simulink library "crm_grc"  (R2024a)
settings: Solver=VariableStepAuto  StartTime=0.0  StopTime=10.0  RelTol=1e-3
undefined symbols (not defined in the file or in its folder): ACRM_Eta_X_rpm, ACRM_MTPAIdGen_X_rpm, ACRM_MTPAIdGen_Y_Nm, ACRM_MTPAIdGenMin_X_rpm, ACRM_MTPAIdGenMin_Y_Nm, ACRM_MTPAIdMot_X_rpm, ACRM_MTPAIdMot_Y_Nm, ACRM_MTPAIdMotMin_X_rpm, ACRM_MTPAIdMotMin_Y_Nm, ACRM_MTPAIqGen_X_rpm, ACRM_MTPAIqGen_Y_Nm, ACRM_MTPAIqGenMin_X_rpm, ACRM_MTPAIqGenMin_Y_Nm, ACRM_MTPAIqMot_X_rpm, ACRM_MTPAIqMot_Y_Nm, ACRM_MTPAIqMotMin_X_rpm, ACRM_MTPAIqMotMin_Y_Nm, ACRM_MTPVIdLimt_X_rpm, DiscIntNeverNeededParam, ENUM_MOTMOD_DISCHARGE, GRC_FAKE_SAMPLE_TIME, KCRM_AtSweep_deg_ovrdflg, KCRM_AtSweep_deg_ovrdval, KCRM_AtSwFWThd_V, KCRM_AtSwStep_ms, KCRM_AtSwThetaStep_deg, KCRM_bRstDebugOverSpd_null, KCRM_BusCurFil_null, KCRM_CurDebugSwt_null, KCRM_CurTqCmdHi_Nm, KCRM_CurTqCmdLo_Nm, KCRM_DcHiBatLDerat_V, KCRM_DcHiBatLLim_V, KCRM_DynoDeratingFiltFac_null, KCRM_FWCEnable_null, KCRM_FWCKi_null, KCRM_FWCKp_null, KCRM_grdIsThetaRampDown_C, KCRM_grdIsThetaRampUp_C, KCRM_IdCmdFilCoeff_null, KCRM_IdCmdMaxLimt_A, KCRM_IdqMapVolHi_V, KCRM_IdqMapVolLo_V, KCRM_IdSp_A_ovrdval, KCRM_IdSpForActvDisc_null, KCRM_IqCmdFilCoeff_null, KCRM_IqDeratingFac_null, KCRM_IqDeratingRecoverTi_ms, KCRM_IqDeratingTi_ms, KCRM_IqDerForFluxWeaken_fac, KCRM_IqSp_A_ovrdval, KCRM_IsSp_A, KCRM_MinVolOfst4FW_V, KCRM_MTPAGenSwitch_flg, KCRM_MTPAMotSwitch_flg, KCRM_MTPVSpdThd_rpm, KCRM_nDebugOverSpd_rpm, KCRM_OCSwFltNormThd_A, KCRM_PILowerLimit_null, KCRM_SpdCtlPrd_s ... (+24)
libraries: GRC_Lib x5, simulink x4
(part 2 of 2)

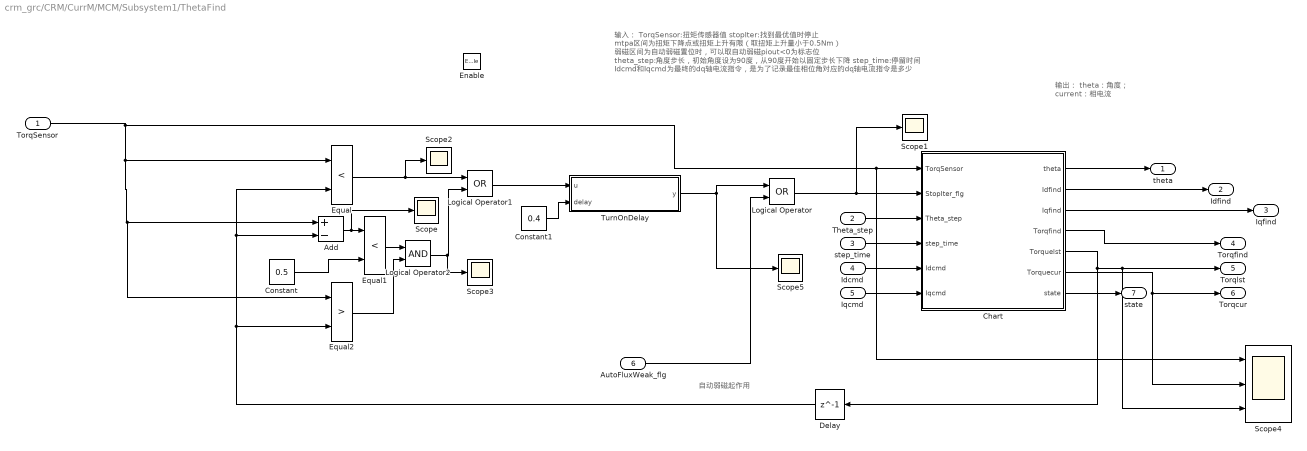
== system crm_grc/CRM/CurrM/MCM/Subsystem1/ThetaFind ==
  note: 输出：
      | theta：角度；
      | current：相电流
  note: 输入：
      | TorqSensor:扭矩传感器值
      | stopIter:找到最优值时停止 mtpa区间为扭矩下降点或扭矩上升有限（取扭矩上升量小于0.5Nm） 弱磁区间为自动弱磁置位时，可以取自动弱磁piout<0为标志位
      | theta_step:角度步长，初始角度设为90度，从90度开始以固定步长下降
      | step_time:停留时间
      | Idcmd和Iqcmd为最终的dq轴电流指令，是为了记录最佳相位角对应的dq轴电流指令是多少
  note: 自动弱磁起作用
  TorqSensor : Inport
  Theta_step : Inport  Port=2
  step_time : Inport  Port=3
  Idcmd : Inport  Port=4
  Iqcmd : Inport  Port=5
  AutoFluxWeak_flg : Inport  Port=6
  Enable : EnablePort  StatesWhenEnabling=reset
  Add : Sum  Inputs=+-
  Chart : Stateflow chart  TreatAsAtomicUnit=on
  Constant : Constant  Value=0.5
  Constant1 : Constant  Value=0.4  OutDataTypeStr=single
  Delay : Delay  DelayLength=1  InputProcessing=Columns as channels (frame based)
  Equal : RelationalOperator  Operator=<  OutDataTypeStr=boolean  RndMeth=Simplest  InputSameDT=off
  Equal1 : RelationalOperator  Operator=<  OutDataTypeStr=boolean  RndMeth=Simplest  InputSameDT=off
  Equal2 : RelationalOperator  Operator=>  OutDataTypeStr=boolean  RndMeth=Simplest  InputSameDT=off
  Logical Operator : Logic  Operator=OR  AllPortsSameDT=off  OutDataTypeStr=boolean
  Logical Operator1 : Logic  Operator=OR  AllPortsSameDT=off  OutDataTypeStr=boolean
  Logical Operator2 : Logic  AllPortsSameDT=off  OutDataTypeStr=boolean
  Scope{,1..3,5} (5 alike) : Scope
  Scope4 : Scope  NumInputPorts=3
  TurnOnDelay : Subsystem  AncestorBlock=Legion_lib/Logic Blocks/TurnOnDelay
      mask Display:
      | color('red');
      | disp('Turn On Delay')
  theta : Outport  VectorParamsAs1DForOutWhenUnconnected=off
  Idfind : Outport  Port=2  VectorParamsAs1DForOutWhenUnconnected=off
  Iqfind : Outport  Port=3  VectorParamsAs1DForOutWhenUnconnected=off
  Torqfind : Outport  Port=4  VectorParamsAs1DForOutWhenUnconnected=off
  Torqlst : Outport  Port=5  VectorParamsAs1DForOutWhenUnconnected=off
  Torqcur : Outport  Port=6  VectorParamsAs1DForOutWhenUnconnected=off
  state : Outport  Port=7  VectorParamsAs1DForOutWhenUnconnected=off
  wires:
  Constant1/1 -> TurnOnDelay/2(delay)
  TurnOnDelay/1(y) -> Logical Operator/1, Scope5/1
  Logical Operator1/1 -> TurnOnDelay/1(u)
  Chart/7(state) -> state/1
  Chart/6(Torquecur) -> Torqcur/1, Scope4/2
  Delay/1 -> Equal/2, Add/2, Equal2/2
  Chart/5(Torquelst) -> Torqlst/1, Scope4/3, Delay/1
  Logical Operator2/1 -> Logical Operator1/2, Scope3/1
  Equal2/1 -> Logical Operator2/2
  Equal1/1 -> Logical Operator2/1
  Constant/1 -> Equal1/2
  Add/1 -> Equal1/1, Scope/1
  Chart/4(Torqfind) -> Torqfind/1
  Equal/1 -> Logical Operator1/1, Scope2/1
  AutoFluxWeak_flg/1 -> Logical Operator/2
  Iqcmd/1 -> Chart/6(Iqcmd)
  Idcmd/1 -> Chart/5(Idcmd)
  Chart/3(Iqfind) -> Iqfind/1
  Chart/2(Idfind) -> Idfind/1
  Chart/1(theta) -> theta/1
  TorqSensor/1 -> Chart/1(TorqSensor), Scope4/1, Add/1, Equal2/1, Equal/1
  Theta_step/1 -> Chart/3(Theta_step)
  Logical Operator/1 -> Chart/2(StopIter_flg), Scope1/1
  step_time/1 -> Chart/4(step_time)

== system crm_grc/CRM/CurrM/MCM/FluxWeaken /PI /Anti-windup ==
  preInt : Inport
  preSat : Inport  Port=2
  Upper Limit : Inport  Port=3
  Lower Limit : Inport  Port=4
  AND3 : Logic  DisableCoverage=on  OutDataTypeStr=boolean
  Constant : Constant  DisableCoverage=on  OutDataTypeStr=int8
  Constant1 : Constant  DisableCoverage=on  Value=0  OutDataTypeStr=Inherit: Inherit via back propagation  PreserveConstantTs=on
  Constant2 : Constant  DisableCoverage=on  Value=-1  OutDataTypeStr=int8
  Constant3 : Constant  DisableCoverage=on  OutDataTypeStr=int8
  Constant4 : Constant  DisableCoverage=on  Value=-1  OutDataTypeStr=int8
  Constant5 : Constant  Value=0  OutDataTypeStr=Inherit: Inherit via back propagation
  Dead Zone Dynamic : simulink/Discontinuities/Dead Zone Dynamic
  Equal1 : RelationalOperator  DisableCoverage=on  Operator===  OutDataTypeStr=boolean  RndMeth=Simplest  InputSameDT=off
  Relational Operator : RelationalOperator  DisableCoverage=on  Operator=~=  OutDataTypeStr=boolean  RndMeth=Simplest  InputSameDT=off
  Relational Operator1 : RelationalOperator  Operator=>  OutDataTypeStr=boolean  RndMeth=Simplest  InputSameDT=off
  Relational Operator2 : RelationalOperator  Operator=>  OutDataTypeStr=boolean  RndMeth=Simplest  InputSameDT=off
  Switch1 : Switch  DisableCoverage=on  Criteria=u2 > Threshold  SaturateOnIntegerOverflow=off  InputSameDT=off
  Switch2 : Switch  DisableCoverage=on  Criteria=u2 > Threshold  SaturateOnIntegerOverflow=off  InputSameDT=off
  Switch3 : Switch  Criteria=u2 ~= 0  RndMeth=Simplest  SaturateOnIntegerOverflow=off  InputSameDT=off
  Out : Outport
  wires:
  Relational Operator2/1 -> Switch2/2
  Constant3/1 -> Switch2/1
  Constant4/1 -> Switch2/3
  AND3/1 -> Switch3/2  "VFWC_IntSat_flg"
  Relational Operator1/1 -> Switch1/2
  Constant2/1 -> Switch1/3
  Dead Zone Dynamic/1 -> Relational Operator/2, Relational Operator1/1
  Upper Limit/1 -> Dead Zone Dynamic/1
  Constant/1 -> Switch1/1
  Switch1/1 -> Equal1/1
  Switch2/1 -> Equal1/2
  Relational Operator/1 -> AND3/1
  preInt/1 -> Switch3/3, Relational Operator2/1
  Switch3/1 -> Out/1
  Constant5/1 -> Relational Operator2/2, Relational Operator1/2, Relational Operator/1
  Equal1/1 -> AND3/2
  preSat/1 -> Dead Zone Dynamic/2
  Lower Limit/1 -> Dead Zone Dynamic/3
  Constant1/1 -> Switch3/1

== system crm_grc/CRM/CurrM/MCM/Subsystem/ThetaFind/TurnOnDelay ==
  u : Inport
  delay : Inport  Port=2
  Data Type Conversion : DataTypeConversion  OutDataTypeStr=single  SaturateOnIntegerOverflow=off  RndMeth=Floor
  sample time : SampleTimeMath  TsampMathOp=Ts Only  weightValue=1  OutDataTypeStr=Inherit: Inherit via back propagation
  turnondelay : Stateflow chart  TreatAsAtomicUnit=on
  y : Outport
  wires:
  sample time/1 -> turnondelay/3(step)
  Data Type Conversion/1 -> sample time/1
  turnondelay/1(y) -> y/1
  delay/1 -> turnondelay/2(delay)
  u/1 -> Data Type Conversion/1, turnondelay/1(u)

== system crm_grc/CRM/CurrM/MCM/Subsystem1/ThetaFind/TurnOnDelay ==
  u : Inport
  delay : Inport  Port=2
  Data Type Conversion : DataTypeConversion  OutDataTypeStr=single  SaturateOnIntegerOverflow=off  RndMeth=Floor
  sample time : SampleTimeMath  TsampMathOp=Ts Only  weightValue=1  OutDataTypeStr=Inherit: Inherit via back propagation
  turnondelay : Stateflow chart  TreatAsAtomicUnit=on
  y : Outport
  wires:
  u/1 -> turnondelay/1(u), Data Type Conversion/1
  delay/1 -> turnondelay/2(delay)
  turnondelay/1(y) -> y/1
  Data Type Conversion/1 -> sample time/1
  sample time/1 -> turnondelay/3(step)

== stateflow chart crm_grc/CRM/CurrM/MCM/Subsystem/ThetaFind/TurnOnDelay/turnondelay ==
  state Off
    en:y=0;
    timer=0;
  state Delay
    en:timer=timer+step;
    du:timer=timer+step;
  state On
    en:y=1;
  (default) -> Off
  (junction 28) -> Off
  (junction 29) -> (junction 28)
  Delay -> Off [order 1] : [~u]
  Off -> (junction 17) : [u]
  (junction 17) -> (junction 24) [order 1] : [timer>=delay-10^-5]
  (junction 17) -> Delay [order 2]
  (junction 24) -> (junction 25)
  Delay -> On [order 2] : [timer>=delay-10^-5]
  On -> (junction 29) : [~u]
  (junction 25) -> On
  data: u input boolean; delay input single; y output boolean =0; timer local single =0; step input single

== stateflow chart crm_grc/CRM/CurrM/MCM/Subsystem1/ThetaFind/Chart ==
  state degression
    en:
    state = 2;
    theta = theta -Theta_step;
  state INIT
    en:
    theta = 80;
    state = 1;
    Torquelst=-5;
    Torquecur=TorqSensor;
  state end
    en:
    state = 4;
    Idfind = Idcmd;
    Iqfind = Iqcmd;
    theta = 90;
    Torqfind=TorqSensor;
  state wait1
    en:
    state = 3;
    du: cnt = cnt + 1;
  (default) -> INIT
  INIT -> degression
  degression -> wait1 : [theta >=0]{cnt = 0;}
  wait1 -> degression [order 2] : [cnt >= step_time]{cnt = 0;Torquecur=TorqSensor;Torquelst=Torquecur;}
  wait1 -> end [order 1] : [StopIter_flg]
  data: TorqSensor input; StopIter_flg input; Theta_step input; cnt local int32; theta output; step_time input; Idcmd input; Idfind output; Iqfind output; Torqfind output; Torquelst output; Iqcmd input; Torquecur output; state output int8

== stateflow chart crm_grc/CRM/CurrM/MCM/Subsystem1/ThetaFind/TurnOnDelay/turnondelay ==
  state Off
    en:y=0;
    timer=0;
  state Delay
    en:timer=timer+step;
    du:timer=timer+step;
  state On
    en:y=1;
  (default) -> Off
  (junction 28) -> Off
  (junction 29) -> (junction 28)
  Delay -> Off [order 1] : [~u]
  Off -> (junction 17) : [u]
  (junction 17) -> (junction 24) [order 1] : [timer>=delay-10^-5]
  (junction 17) -> Delay [order 2]
  (junction 24) -> (junction 25)
  Delay -> On [order 2] : [timer>=delay-10^-5]
  On -> (junction 29) : [~u]
  (junction 25) -> On
  data: u input boolean; delay input single; y output boolean =0; timer local single =0; step input single

== stateflow chart crm_grc/CRM/CurrM/MCM/IArb ==
  settings: description=$TL$ stepfunctionclass=GlobalFunctionClasses/INLINE_FCN; $TL$
  (default) -> (junction 32)
  (junction 32) -> (junction 35) [order 1] : [ActvDichEna_flg]
  (junction 32) -> (junction 11) [order 2]
  (junction 35) -> (junction 36) : {
      |   IdCmd = IdCmdForActvDich_A;
      |   IqCmd = 0;
      |  }
  (junction 11) -> (junction 12) [order 1] : [CurSpEna_flg]
  (junction 11) -> (junction 14) [order 2]
  (junction 12) -> (junction 13) : {
      |   IdCmd = IdSpAct;
      |   IqCmd = IqSpAct;
      |  }
  (junction 14) -> (junction 15) [order 1] : [CurLoopEna_flg]
  (junction 14) -> (junction 17) [order 2] : {
      |   IdCmd = 0;
      |   IqCmd = 0;
      |  }
  (junction 15) -> (junction 16) : {
      |   IdCmd = IdRef;
      |   IqCmd = IqRef;
      |  }
  (junction 16) -> (junction 17)
  (junction 13) -> (junction 16)
  (junction 36) -> (junction 13)
  (junction 17) -> (junction 18)
  data: IdRef input; IqRef input; IdSpAct input; IqSpAct input; CurLoopEna_flg input; IdCmd output single; IqCmd output single; CurSpEna_flg input boolean; ActvDichEna_flg input boolean; IdCmdForActvDich_A input single
  data IdRef settings: description=|
      | Current reference of d axis deduced by T-n
      | $TL$ variable=GLOBAL/LocalVariables/TM/Current/Id_Ref; $TL$
  data IqRef settings: description=|
      | Current reference of q axis deduced by T-n
      | $TL$ variable=GLOBAL/LocalVariables/TM/Current/Iq_Ref; $TL$
  data IdSpAct settings: description=|
      | Current setpoint of d axis
      | $TL$ variable=GLOBAL/GlobalVariables/MCU/Function/TM/APPL_TM_Id_Setp; $TL$
  data IqSpAct settings: description=|
      | Current setpoint of q axis
      | 
      | $TL$ variable=GLOBAL/GlobalVariables/MCU/Function/TM/APPL_TM_Iq_Setp; $TL$
  data CurLoopEna_flg settings: description=|
      | Control mode of TM controller, 0 for Voltage loop, 1 for Current loop, 2 for Torque loop, 3 for Speed loop
      | $TL$ variable=GLOBAL/GlobalVariables/MCU/Function/TM/ECUL_TM_Ctrl_Mod; $TL$
  data IdCmd settings: description=|
      | Current command of d axis
      | $TL$ variable=GLOBAL/LocalVariables/TM/Current/Id_Cmd; $TL$
  data IqCmd settings: description=|
      | Current command of q axis
      | $TL$ variable=GLOBAL/LocalVariables/TM/Current/Iq_Cmd; $TL$

== stateflow chart crm_grc/CRM/CurrM/MCM/Subsystem/ThetaFind/Chart ==
  state degression
    en:
    state = 2;
    theta = theta -Theta_step;
  state INIT
    en:
    theta = KMCM_AtSwInitPos_deg;
    state = 1;
    Torquelst=-5;
    Torquecur=TorqSensor;
  state end
    en:
    state = 4;
    Idfind = Idcmd;
    Iqfind = Iqcmd;
    theta = KMCM_AtSwInitPos_deg;
    Torqfind=TorqSensor;
  state wait1
    en:
    state = 3;
    du: cnt = cnt + 1;
  (default) -> INIT
  INIT -> degression
  degression -> wait1 : [theta >=0]{cnt = 0;}
  wait1 -> degression [order 1] : [cnt >= step_time]{cnt = 0;Torquecur=TorqSensor;Torquelst=Torquecur;}
  wait1 -> end [order 2] : [StopIter_flg]
  data: TorqSensor input; StopIter_flg input; Theta_step input; theta output; step_time input; Idcmd input; Idfind output; Iqfind output; Torqfind output; Torquelst output; Iqcmd input; Torquecur output; state output int8; cnt local int32 =0; KMCM_AtSwInitPos_deg parameter
